simulink model "RobustInverseDynamicsControl"  (R2021a)
settings: Solver=FixedStepAuto  StartTime=0.0  StopTime=5  FixedStep=0.0001  RelTol=1e-3
InitFcn:
  | kd1 = 100;
  | kd2 = 100;
  | kd3 = 100;
  | kp1 = 100;
  | kp2 = 100;
  | kp3 = 100;
settings Model: Creator=negin  LastModifiedBy=negin

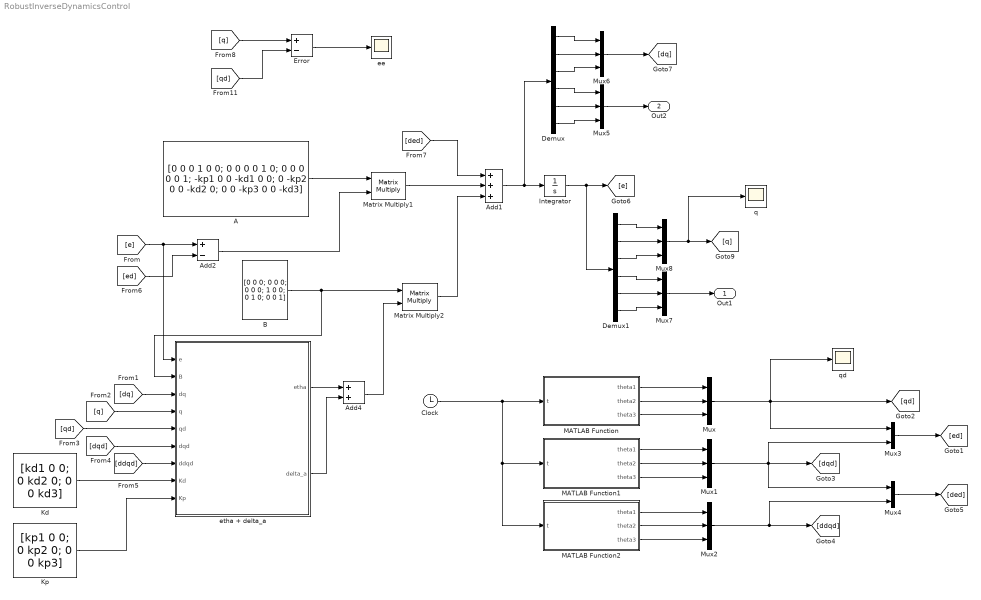
== system RobustInverseDynamicsControl ==
  A : Constant  Value=[0 0 0 1 0 0; 0 0 0 0 1 0; 0 0 0 0 0 1; -kp1 0 0 -kd1 0 0; 0 -kp2 0 0 -kd2 0; 0 0 -kp3 0 0 -kd3]  VectorParams1D=off
  Add1 : Sum  Inputs=+++
  Add2 : Sum  Inputs=+-
  Add4 : Sum
  B : Constant  Value=[0 0 0; 0 0 0; 0 0 0; 1 0 0; 0 1 0; 0 0 1]  VectorParams1D=off
  Clock : Clock
      settings: Decimation=5
  Demux : Demux  Outputs=6
  Demux1 : Demux  Outputs=6
  Error : Sum  Inputs=+-
  Integrator : Integrator  InitialCondition=10^-4*[1 1 1 1 1 1]
  Kd : Constant  Value=[kd1 0 0; 0 kd2 0; 0 0 kd3]  VectorParams1D=off
  Kp : Constant  Value=[kp1 0 0; 0 kp2 0; 0 0 kp3]  VectorParams1D=off
  MATLAB Function : MATLAB Function  TreatAsAtomicUnit=on
  MATLAB Function1 : MATLAB Function  TreatAsAtomicUnit=on
  MATLAB Function2 : MATLAB Function  TreatAsAtomicUnit=on
  Matrix Multiply1 : Product  Multiplication=Matrix(*)
  Matrix Multiply2 : Product  Multiplication=Matrix(*)
  Mux{,1..2,5..8} (7 alike) : Mux  Inputs=3
  Mux3 : Mux  Inputs=2
  Mux4 : Mux  Inputs=2
  ee : Scope
  etha + delta_a : MATLAB Function  TreatAsAtomicUnit=on
  q : Scope
  qd : Scope
  Out1 : Outport
  Out2 : Outport  Port=2
  wires:
  MATLAB Function/1(theta1) -> Mux/1
  Clock/1 -> MATLAB Function/1(t), MATLAB Function1/1(t), MATLAB Function2/1(t)
  MATLAB Function/2(theta2) -> Mux/2
  MATLAB Function/3(theta3) -> Mux/3
  Mux/1 -> qd/1, [qd], Mux3/1
  MATLAB Function1/1(theta1) -> Mux1/1
  MATLAB Function1/2(theta2) -> Mux1/2
  MATLAB Function1/3(theta3) -> Mux1/3
  MATLAB Function2/1(theta1) -> Mux2/1
  MATLAB Function2/2(theta2) -> Mux2/2
  MATLAB Function2/3(theta3) -> Mux2/3
  Mux1/1 -> [dqd], Mux4/1, Mux3/2
  Mux2/1 -> [ddqd], Mux4/2
  A/1 -> Matrix Multiply1/1
  B/1 -> etha + delta_a/2(B), Matrix Multiply2/1
  Mux3/1 -> [ed]
  [e] -> etha + delta_a/1(e), Add2/1
  [ed] -> Add2/2
  Add2/1 -> Matrix Multiply1/2
  Matrix Multiply2/1 -> Add1/3
  Matrix Multiply1/1 -> Add1/2
  Mux4/1 -> [ded]
  [ded] -> Add1/1
  Add1/1 -> Demux/1, Integrator/1
  Integrator/1 -> Demux1/1, [e]
  Demux/4 -> Mux5/1
  Demux/5 -> Mux5/2
  Demux/6 -> Mux5/3
  Demux/1 -> Mux6/1
  Demux/2 -> Mux6/2
  Demux/3 -> Mux6/3
  Mux6/1 -> [dq]
  Mux5/1 -> Out2/1
  Demux1/4 -> Mux7/1
  Mux8/1 -> q/1, [q]
  Demux1/5 -> Mux7/2
  Demux1/3 -> Mux8/3
  Demux1/2 -> Mux8/2
  Demux1/6 -> Mux7/3
  Mux7/1 -> Out1/1
  Demux1/1 -> Mux8/1
  [q] -> Error/1
  [qd] -> Error/2
  Error/1 -> ee/1
  etha + delta_a/1(etha) -> Add4/1
  etha + delta_a/2(delta_a) -> Add4/2
  Add4/1 -> Matrix Multiply2/2
  [dq] -> etha + delta_a/3(dq)
  [q] -> etha + delta_a/4(q)
  [qd] -> etha + delta_a/5(qd)
  [dqd] -> etha + delta_a/6(dqd)
  [ddqd] -> etha + delta_a/7(ddqd)
  Kd/1 -> etha + delta_a/8(Kd)
  Kp/1 -> etha + delta_a/9(Kp)

== matlab function RobustInverseDynamicsControl/MATLAB Function ==
  data: theta1 output; t input; theta2 output; theta3 output
function [theta1, theta2, theta3] = desiredTraj(t)
theta1 = 0.1309*t^2 + 0.0147*t^3 - 0.0085*t^4 + 0.0007*t^5;
theta2 = 0.1309*t^2 - 0.0188*t^3 - 0.001*t^4 + 0.0002*t^5;
theta3 = 0.1309*t^2 + 0.0314*t^3 - 0.0123*t^4 + 0.001*t^5;

== matlab function RobustInverseDynamicsControl/etha + delta_a ==
  data: e input; etha output; B input; dq input; q input; qd input; dqd input; ddqd input; delta_a output; Kd input; Kp input
function [etha, delta_a] = etha_deltaA(e, B, dq, q, qd, dqd, ddqd, Kd, Kp)

m1 = 1;
m2 = 1;
m3 = 1;

l1 = 1;
l2 = 1;
l3 = 1;

r1 = l1/2;
r2 = l2/2;
r3 = l3/2;

R1 = 0.05;
R2 = 0.05;
R3 = 0.05;

g = 9.81;

a1 = m2*r2^2 + m3*l2^2;
a2 = m3*r3^2;
a3 = m3*r3*l2;
b1 = (m2*r2 + m3*l2)*g;
b2 = m3*r3*g;
I1 = 0.5*m1*R1^2;
I2 = 0.5*m2*R2^2;
I3 = 0.5*m3*R3^2;

M11 = a1*cos(q(2))^2 + a2*cos(q(2) + q(3))^2 + 2*a3*cos(q(2))*cos(q(2) + q(3)) + I1;
M12 = 0; 
M13 = 0; 
M21 = 0; 
M31 = 0;
M22 = a1 + a2 + 2*a3*cos(q(3)) + I2;
M23 = a2 + a3*cos(q(3));
M32 = a2 + a3*cos(q(3));
M33 = a2 + I3;
M = [M11 M12 M13; M21 M22 M23; M31 M32 M33];

C11 = -0.5*a1*dq(2)*sin(2*q(2)) - 0.5*a2*(dq(2) + dq(3))*sin(2*q(2) + 2*q(3))...
    - a3*dq(2)*sin(2*q(2) + q(3)) - a3*dq(3)*cos(q(2))*sin(q(2) + q(3));
C12 = -0.5*a1*dq(1)*sin(2*q(2)) - 0.5*a2*dq(1)*sin(2*q(2) + 2*q(3)) - ...
    a3*dq(1)*sin(2*q(2) + q(3));
C13 = -0.5*a2*dq(1)*sin(2*q(2) + 2*q(3)) - a3*dq(1)*cos(q(2))*sin(q(2) + q(3));
C21 = -C12;
C22 = -a3*dq(3)*sin(q(3));
C23 = -a3*(dq(2) + dq(3))*sin(q(3));
C31 = -C13;
C32 = a3*dq(2)*sin(q(3));
C33 = 0;
C = [C11 C12 C13; C21 C22 C23; C31 C32 C33];

G11 = 0;
G21 = m2*l2*sin(q(2))*g/2 - m3*l3*sin(q(2) + q(3))*g/2 - m3*l2*sin(q(2))*g;
G31 = -m3*l3*sin(q(2) + q(3))*g/2;
G = [G11; G21; G31];

P = [-49 0 0 53 0 0; 0 -49 0 0 53 0; 0 0 -49 0 0 53; 53 0 0 -59 0 0; 0 53 0 0 -59 0; 0 0 53 0 0 -59];
Rho = 0.01;

Mhat = [3.5 0 0; 0 3.5 0.75; 0 0.75 1.25];
Chat = [2 1.25 1; -1.25 0.5 0.5; -1 0.5 0];
Ghat = [0; 20; 5];

epsilon = 0.1;
con = abs(transpose(B)*P*e);
consize = sqrt(con(1)^2 + con(2)^2 + con(3)^2);
if consize > epsilon
    delta_a = -(Rho/consize).*transpose(B)*P*e;
else
    delta_a = -(Rho/epsilon).*transpose(B)*P*e;
end

aq = ddqd - Kd*(q - qd) - Kp*(dq - dqd) + delta_a;

etha = inv(M)*((-M + Mhat)*aq + (-C + Chat)*dq + (-G + Ghat));

end

== matlab function RobustInverseDynamicsControl/MATLAB Function1 ==
  data: theta1 output; t input; theta2 output; theta3 output
function [theta1, theta2, theta3] = ddesiredTraj(t)
theta1 = 0.1309*2*t + 0.0147*3*t^2 - 0.0085*4*t^3 + 0.0007*5*t^4;
theta2 = 0.1309*2*t - 0.0188*3*t^2 - 0.001*4*t^3 + 0.0002*5*t^4;
theta3 = 0.1309*2*t + 0.0314*3*t^2 - 0.0123*4*t^3 + 0.001*5*t^4;

== matlab function RobustInverseDynamicsControl/MATLAB Function2 ==
  data: theta1 output; t input; theta2 output; theta3 output
function [theta1, theta2, theta3] = dddesiredTraj(t)
theta1 = 0.1309*2 + 0.0147*3*2*t - 0.0085*4*3*t^2 + 0.0007*5*4*t^3;
theta2 = 0.1309*2 - 0.0188*3*2*t - 0.001*4*3*t^2 + 0.0002*5*4*t^3;
theta3 = 0.1309*2 + 0.0314*3*2*t - 0.0123*4*3*t^2 + 0.001*5*4*t^3;
